simulink model "DR_Smart_Triage"  (R2026a)
settings: Solver=VariableStepAuto
libraries: simulink x2

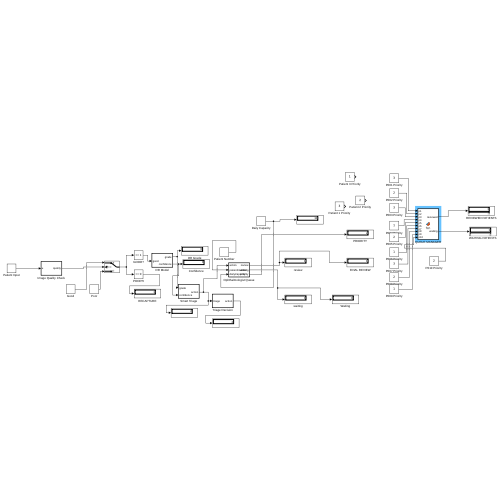
[thumbnail: Simulink's stored preview of the top-level diagram]
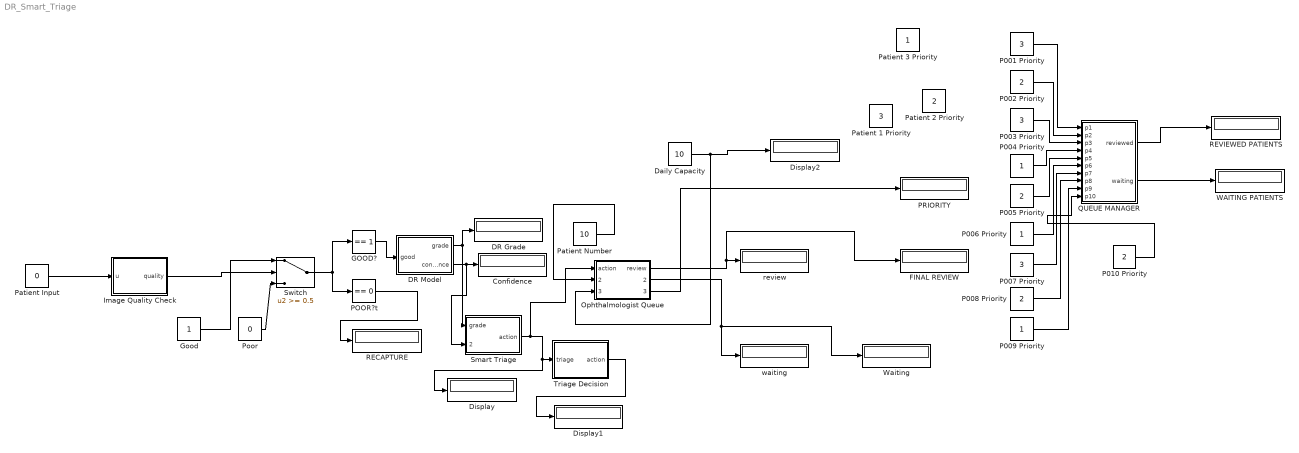
== system DR_Smart_Triage ==
  Confidence : Display
  DR Grade : Display
  DR Model : MATLAB Function  TreatAsAtomicUnit=on
  Daily Capacity : Constant  Value=10
  Display : Display
  Display1 : Display
  Display2 : Display
  FINAL REVIEW : Display
  GOOD? : simulink/Logic and Bit Operations/Compare To Constant  relop===  const=1  OutDataTypeStr=boolean
  Good : Constant
  Image Quality Check : MATLAB Function  TreatAsAtomicUnit=on
  Ophthalmologist Queue : MATLAB Function  TreatAsAtomicUnit=on
  P001 Priority : Constant  Value=3
  P002 Priority : Constant  Value=2
  P003 Priority : Constant  Value=3
  P004 Priority : Constant
  P005 Priority : Constant  Value=2
  P006 Priority : Constant
  P007 Priority : Constant  Value=3
  P008 Priority : Constant  Value=2
  P009 Priority : Constant
  P010 Priority : Constant  Value=2
  POOR?t : simulink/Logic and Bit Operations/Compare To Constant  relop===  const=0  OutDataTypeStr=boolean
  PRIORITY : Display
  Patient 1 Priority : Constant  Value=3
  Patient 2 Priority : Constant  Value=2
  Patient 3 Priority : Constant
  Patient Input : Constant  Value=0
  Patient Number : Constant  Value=10
  Poor : Constant  Value=0
  QUEUE MANAGER : MATLAB Function  TreatAsAtomicUnit=on
  RECAPTURE : Display
  REVIEWED PATIENTS : Display
  Smart Triage : MATLAB Function  TreatAsAtomicUnit=on
  Switch : Switch  Threshold=0.5  SaturateOnIntegerOverflow=off  InputSameDT=off
  Triage Decision : MATLAB Function  TreatAsAtomicUnit=on
  WAITING PATIENTS : Display
  Waiting : Display
  review : Display
  waiting : Display
  wires:
  Patient Input/1 -> Image Quality Check/1(u)
  Image Quality Check/1(quality) -> Switch/2
  Good/1 -> Switch/1
  Poor/1 -> Switch/3
  Switch/1 -> POOR?t/1, GOOD?/1
  GOOD?/1 -> DR Model/1(good)
  POOR?t/1 -> RECAPTURE/1
  DR Model/1(grade) -> DR Grade/1, Smart Triage/1(grade)
  DR Model/2(confidence) -> Smart Triage/2(confidence), Confidence/1
  Smart Triage/1(action) -> Ophthalmologist Queue/1(action), Display/1, Triage Decision/1(triage)
  Triage Decision/1(action) -> Display1/1
  Patient Number/1 -> Ophthalmologist Queue/2(patientNumber)
  Ophthalmologist Queue/1(review) -> FINAL REVIEW/1, review/1
  Ophthalmologist Queue/2(waiting) -> waiting/1, Waiting/1
  Daily Capacity/1 -> Ophthalmologist Queue/3(dailyCapacity), Display2/1
  Ophthalmologist Queue/3(priority) -> PRIORITY/1
  P001 Priority/1 -> QUEUE MANAGER/1(p1)
  P002 Priority/1 -> QUEUE MANAGER/2(p2)
  P003 Priority/1 -> QUEUE MANAGER/3(p3)
  P004 Priority/1 -> QUEUE MANAGER/4(p4)
  P005 Priority/1 -> QUEUE MANAGER/5(p5)
  P006 Priority/1 -> QUEUE MANAGER/6(p6)
  P007 Priority/1 -> QUEUE MANAGER/7(p7)
  P008 Priority/1 -> QUEUE MANAGER/8(p8)
  P009 Priority/1 -> QUEUE MANAGER/9(p9)
  P010 Priority/1 -> QUEUE MANAGER/10(p10)
  QUEUE MANAGER/2(waiting) -> WAITING PATIENTS/1
  QUEUE MANAGER/1(reviewed) -> REVIEWED PATIENTS/1

== matlab function DR_Smart_Triage/DR Model ==
  data: good input; grade output; confidence output
function [grade, confidence] = fcn(good)
%#codegen

if good == 1
    grade = 2;
    confidence = 90;
else
    grade = 0;
    confidence = 0;
end

== matlab function DR_Smart_Triage/Image Quality Check ==
  data: u input; quality output
function quality = fcn(u)
%#codegen

if u >= 0.5
    quality = 1;     % GOOD
else
    quality = 0;     % POOR
end

== matlab function DR_Smart_Triage/Smart Triage ==
  data: grade input; action output; confidence input
function action = fcn(grade, confidence)
%#codegen

if confidence < 80
    action = 2;

elseif grade >= 3
    action = 3;

elseif grade >= 1
    action = 2;

else
    action = 1;
end

== matlab function DR_Smart_Triage/Triage Decision ==
  data: triage input; action output
function action = fcn(triage)
%#codegen

if triage == 1
    action = 1;
elseif triage == 2
    action = 2;
else
    action = 3;
end

== matlab function DR_Smart_Triage/Ophthalmologist Queue ==
  data: action input; review output; patientNumber input; waiting output; dailyCapacity input; priority output
function [review, waiting, priority] = fcn(action, patientNumber, dailyCapacity)
%#codegen

if action == 3
    priority = 3;
elseif action == 2
    priority = 2;
else
    priority = 1;
end

if action == 1
    review = 0;
    waiting = 0;
elseif patientNumber <= dailyCapacity
    review = 1;
    waiting = 0;
else
    review = 0;
    waiting = 1;
end

== matlab function DR_Smart_Triage/QUEUE MANAGER ==
  data: p1 input; reviewed output; p2 input; p3 input; p4 input; p5 input; p6 input; p7 input; p8 input; p9 input; p10 input; waiting output
function [reviewed, waiting] = fcn(p1,p2,p3,p4,p5,p6,p7,p8,p9,p10)
%#codegen

DailyCapacity = 10;

priority = [p1 p2 p3 p4 p5 p6 p7 p8 p9 p10];

% Sort patients from highest to lowest priority
[~, order] = sort(priority,'descend');

% Number of patients reviewed
reviewed = min(DailyCapacity, length(priority));

% Remaining patients waiting
waiting = length(priority) - reviewed;

end
